simulink model "simulatoreBP"  (R2024b)
settings: Solver=VariableStepAuto  StartTime=0.0  StopTime=20  RelTol=1e-3
undefined symbols (not defined in the file): d_sinewave_amplitude, d_sinewave_frequency_Hz, d_sinewave_phase_rad, d_step_amplitude, d_step_time, dt, f_inf_rads, makeweight, power_v_noise, reference_step_amplitude, reference_step_time, tol_mm
libraries: cstblocks x3, simulink x1
settings Model: Creator=USER  LastModifiedBy=USER
settings SolverCC: AlgebraicLoopSolver=TrustRegion
settings DebuggingCC: UnconnectedInputMsg=warning  UnconnectedOutputMsg=warning  UnconnectedLineMsg=warning
settings ModelReferenceCC: EnableRefExpFcnMdlSchedulingChecks=on
settings RTWCC: GPUComputeCapability=3.5  DLArmComputeVersion=19.05

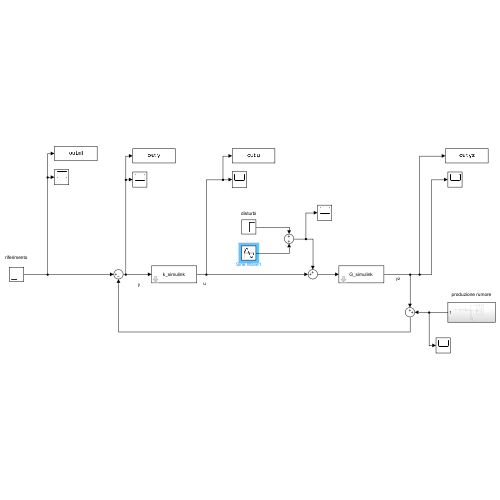
[thumbnail: Simulink's stored preview of the top-level diagram]
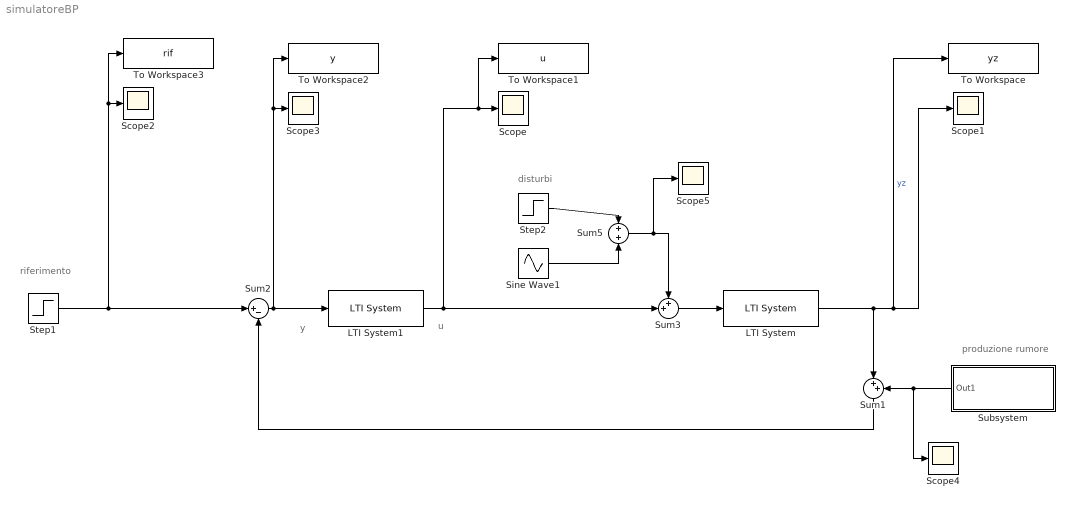
== system simulatoreBP ==
  note: produzione rumore
  note: riferimento
  note: u
  note: y
  note: disturbi
  LTI System : cstblocks/LTI System  sys=G_simulink  IC=[0]  PadeOrder=0
  LTI System1 : cstblocks/LTI System  sys=k_simulink  IC=[]  PadeOrder=0
  Scope{,1..5} (6 alike) : Scope
  Sine Wave1 : Sin  Amplitude=d_sinewave_amplitude  Frequency=2*pi*d_sinewave_frequency_Hz  Phase=d_sinewave_phase_rad  SampleTime=0
  Step1 : Step  Time=reference_step_time  After=reference_step_amplitude  SampleTime=0
  Step2 : Step  Time=d_step_time  After=d_step_amplitude  SampleTime=0
  Subsystem : Subsystem
  Sum1 : Sum  Inputs=|++
  Sum2 : Sum  Inputs=|+-
  Sum3 : Sum  Inputs=++|
  Sum5 : Sum
  To Workspace : ToWorkspace  VariableName=yz  SaveFormat=Timeseries  SampleTime=-1
  To Workspace1 : ToWorkspace  VariableName=u  SaveFormat=Timeseries  SampleTime=-1
  To Workspace2 : ToWorkspace  VariableName=y  SaveFormat=Timeseries  SampleTime=-1
  To Workspace3 : ToWorkspace  VariableName=rif  SaveFormat=Timeseries  SampleTime=-1
  wires:
  LTI System/1 -> Scope1/1, To Workspace/1, Sum1/1  "yz"
  LTI System1/1 -> Sum3/2, To Workspace1/1, Scope/1
  Sum2/1 -> LTI System1/1, To Workspace2/1, Scope3/1
  Sum1/1 -> Sum2/2
  Sum3/1 -> LTI System/1
  Step1/1 -> Sum2/1, To Workspace3/1, Scope2/1
  Step2/1 -> Sum5/1
  Sine Wave1/1 -> Sum5/2
  Sum5/1 -> Scope5/1, Sum3/1
  Subsystem/1(Out1) -> Scope4/1, Sum1/2

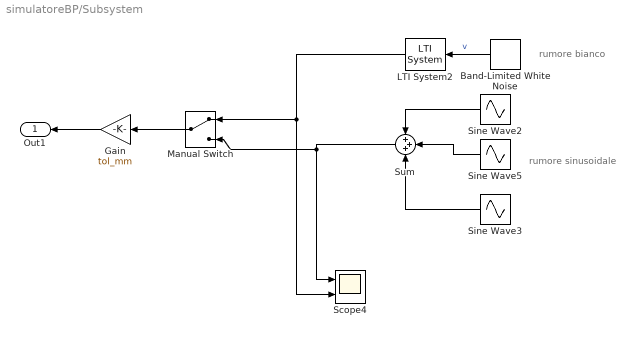
== system simulatoreBP/Subsystem ==
  note: rumore sinusoidale
  note: rumore bianco
  Band-Limited White Noise : simulink/Sources/Band-Limited White Noise  Cov=power_v_noise  Ts=dt  seed=[23341]
  Gain : Gain  Gain=tol_mm
  LTI System2 : cstblocks/LTI System  sys=makeweight(0, [f_inf_rads sqrt(2)/2], 1)  IC=[]  PadeOrder=0
  Manual Switch : ManualSwitch
  Scope4 : Scope  NumInputPorts=2
  Sine Wave2 : Sin  Amplitude=power_v_noise * 10^6 * rand  Frequency=f_inf_rads + (2*f_inf_rads - f_inf_rads) * rand;  Phase=2*pi*rand  SampleTime=0
  Sine Wave3 : Sin  Amplitude=power_v_noise * 10^6 * rand  Frequency=f_inf_rads + (2*f_inf_rads - f_inf_rads) * rand;  Phase=2*pi*rand  SampleTime=0
  Sine Wave5 : Sin  Amplitude=power_v_noise * 10^6 * rand  Frequency=f_inf_rads + (2*f_inf_rads - f_inf_rads) * rand;  Phase=2*pi*rand  SampleTime=0
  Sum : Sum  Inputs=+++
  Out1 : Outport
  wires:
  Sine Wave2/1 -> Sum/1
  Sine Wave3/1 -> Sum/3
  Sine Wave5/1 -> Sum/2
  Band-Limited White Noise/1 -> LTI System2/1  "v"
  Sum/1 -> Manual Switch/2, Scope4/1
  LTI System2/1 -> Manual Switch/1, Scope4/2
  Manual Switch/1 -> Gain/1
  Gain/1 -> Out1/1
